simulink model "untitled"  (R2018a)
settings: Solver=ode4  StartTime=0.0  StopTime=50  FixedStep=0.04  RelTol=1e-3
settings Model: SimulationMode=accelerator  Creator=Hungs  LastModifiedBy=Hungs
settings DataIOCC: SaveTime=off
settings OptimizationCC: EfficientMapNaN2IntZero=off
settings HardwareCC: TargetBitPerPointer=64  TargetBitPerSizeT=64  TargetBitPerPtrDiffT=64  TargetLongLongMode=on  TargetIntDivRoundTo=Zero  TargetEndianess=LittleEndian  TargetWordSize=64  TargetHWDeviceType=MATLAB Host  ProdEqTarget=off
settings CodeAppCC: MaxIdLength=128
settings GRTTargetCC: TargetLangStandard=C89/C90 (ANSI)  CombineOutputUpdateFcns=off  GRTInterface=on

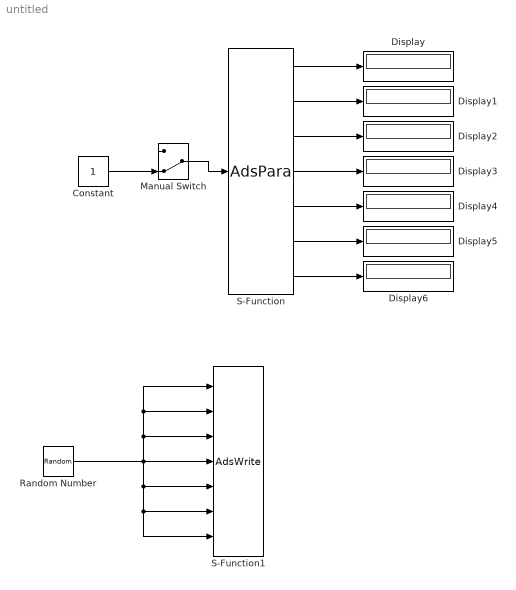
== system untitled ==
  Constant : Constant
  Display{,1..6} (7 alike) : Display
  Manual Switch : ManualSwitch  CurrentSetting=0
  Random Number : RandomNumber  Mean=10  Variance=5
  S-Function : S-Function  FunctionName=AdsPara  Parameters=[192 168 56 1 1 1] 851  SFunctionDeploymentMode=off  EnableBusSupport=off
  S-Function1 : S-Function  FunctionName=AdsWrite  SFunctionDeploymentMode=off  EnableBusSupport=off
  wires:
  S-Function/1 -> Display/1
  S-Function/2 -> Display1/1
  S-Function/3 -> Display2/1
  S-Function/5 -> Display4/1
  S-Function/4 -> Display3/1
  S-Function/6 -> Display5/1
  S-Function/7 -> Display6/1
  Constant/1 -> Manual Switch/2
  Manual Switch/1 -> S-Function/1
  Random Number/1 -> S-Function1/3, S-Function1/2, S-Function1/1, S-Function1/4, S-Function1/6, S-Function1/7, S-Function1/5
